simulink model "AOO_group11"  (R2023a)
settings: Solver=FixedStepAuto  StartTime=0.0  StopTime=10.0  FixedStep=1e-3  RelTol=1e-3  EnableMultiTasking=on
undefined symbols (not defined in the file): D10, D11, D2, D4, D5, D8, PTA0, PTA2, PTB23, PTB9, PTD0, PTD2
libraries: frdmk64flib x8
settings Model: ExtModeTrigDuration=5  Creator=faraa  LastModifiedBy=faraa
settings OptimizationCC: EnhancedBackFolding=on  PassReuseOutputArgsAs=Individual arguments  ZeroExternalMemoryAtStartup=off  ZeroInternalMemoryAtStartup=off  MaxStackSize=64  OptimizeBlockOrder=speed  DifferentSizesBufferReuse=on  OptimizationCustomize=off  EfficientTunableParamExpr=on
settings DebuggingCC: ParameterTunabilityLossMsg=error
settings HardwareCC: ProdBitPerPointer=32  ProdBitPerSizeT=32  ProdBitPerPtrDiffT=32  ProdLargestAtomicInteger=Long  ProdLargestAtomicFloat=Double  ProdWordSize=32  ProdHWDeviceType=ARM Compatible->ARM Cortex
settings SFSimCC: MATLABDynamicMemAlloc=off
settings RTWCC: Description=Embedded Coder  SystemTargetFile=ert.tlc  HardwareBoard=NXP FRDM-K64F  TLCOptions="-aInlineSetEventsForThisBaseRateFcn=TLC_FALSE -aSuppressMultiTaskScheduler=TLC_FALSE  -aRateBasedStepFcn=0"  TemplateMakefile=ert_default_tmf  Toolchain=GNU Tools for ARM Embedded Processors
settings CodeAppCC: ForceParamTrailComments=on  IgnoreCustomStorageClasses=off  OperatorAnnotations=on  SimulinkDataObjDesc=on  SFDataObjDesc=on  InsertBlockDesc=on
settings ERTTargetCC: ExtModeTransport=4  ExtModeMexFile=sendToCommService

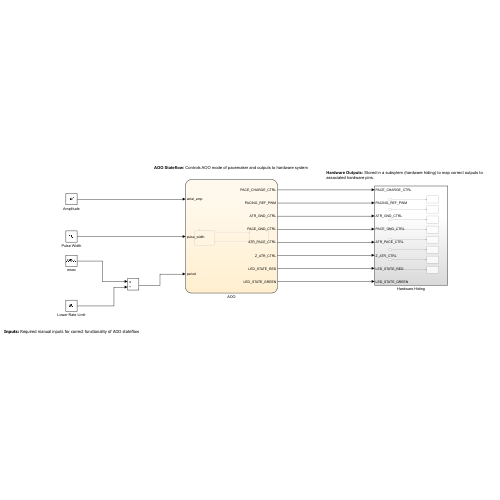
[thumbnail: Simulink's stored preview of the top-level diagram]
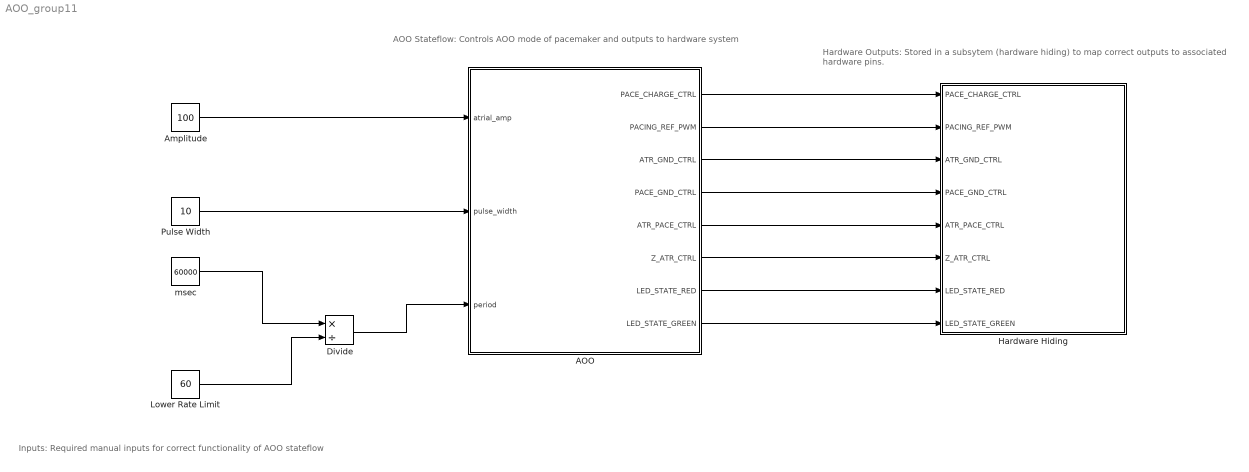
== system AOO_group11 ==
  note: Inputs: Required manual inputs for correct functionality of AOO stateflow
  note: Hardware Outputs: Stored in a subsytem (hardware hiding) to map correct outputs to associated hardware pins.
  note: AOO Stateflow: Controls AOO mode of pacemaker and outputs to hardware system
  AOO : Stateflow chart  TreatAsAtomicUnit=on
      settings: PortSchema="{\"entries\":[{\"content\":{\"sides\":[{\"content\":{\"connectorIds\":[\"In1\",\"In2\",\"In3\"]},\"type\":\"ConnectorPlacement.EquallySpacedRectSide\",\"uuid\":\"95ae3ac6-e5ac-4d1d-8671-90628795223e\"},{\"content\":{\"connectorIds\":[\"Out1\",\"Out2\",\"Out3\",\"Out4\",\"Out5\",\"Out8\",\"Out6\",\"Out7\"],\"side\":\"RIGHT\"},\"type\":\"ConnectorPlacement.EquallySpacedRectSide\",\"uuid\":\"b0ec74bf-e631-4588-a0db-5024556e9f33\"},{\"content\":{\"side\":\"TOP\"},\"type\":\"ConnectorPlacement.EquallySpacedRectSide\",\"uuid\":\"f45d59e1-716f-4ed7-bde8-ed6d2f349a65\"}]},\"type\":\"ConnectorPlacement.EquallySpacedConnector\",\"uuid\":\"a31986a1-9390-4687-9321-72416b41487c\"}],\"packageUris\":[\"http://schema.mathworks.com/mf0/Connector/R2020b\"],\"version\":\"1.0\"}"
  Amplitude : Constant  Value=100
  Divide : Product  Inputs=*/
  Hardware Hiding : Subsystem
  Lower Rate Limit : Constant  Value=60
  Pulse Width : Constant  Value=10
  msec : Constant  Value=60000
  wires:
  Amplitude/1 -> AOO/1(atrial_amp)
  Pulse Width/1 -> AOO/2(pulse_width)
  msec/1 -> Divide/1
  Lower Rate Limit/1 -> Divide/2
  Divide/1 -> AOO/3(period)
  AOO/1(PACE_CHARGE_CTRL) -> Hardware Hiding/1(PACE_CHARGE_CTRL)
  AOO/2(PACING_REF_PWM) -> Hardware Hiding/2(PACING_REF_PWM)
  AOO/3(ATR_GND_CTRL) -> Hardware Hiding/3(ATR_GND_CTRL)
  AOO/4(PACE_GND_CTRL) -> Hardware Hiding/4(PACE_GND_CTRL)
  AOO/5(ATR_PACE_CTRL) -> Hardware Hiding/5(ATR_PACE_CTRL)
  AOO/8(Z_ATR_CTRL) -> Hardware Hiding/6(Z_ATR_CTRL)
  AOO/6(LED_STATE_RED) -> Hardware Hiding/7(LED_STATE_RED)
  AOO/7(LED_STATE_GREEN) -> Hardware Hiding/8(LED_STATE_GREEN)

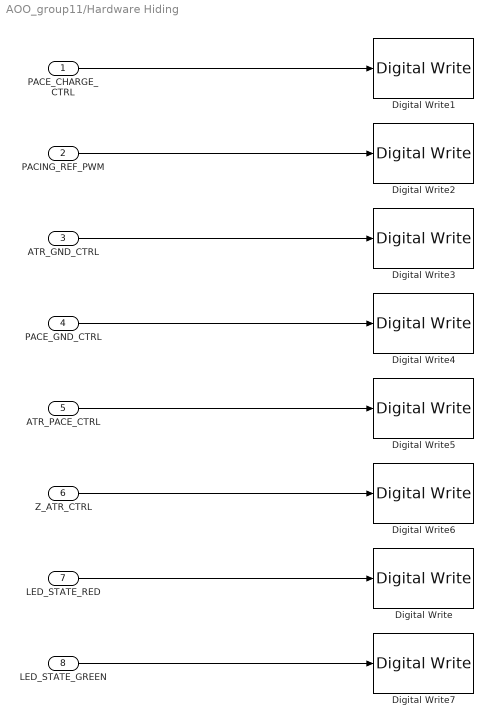
== system AOO_group11/Hardware Hiding ==
  PACE_CHARGE_CTRL : Inport
  PACING_REF_PWM : Inport  Port=2
  ATR_GND_CTRL : Inport  Port=3
  PACE_GND_CTRL : Inport  Port=4
  ATR_PACE_CTRL : Inport  Port=5
  Z_ATR_CTRL : Inport  Port=6
  LED_STATE_RED : Inport  Port=7
  LED_STATE_GREEN : Inport  Port=8
  Digital Write : frdmk64flib/Digital Write  Whichpin=RED_LED
  Digital Write1 : frdmk64flib/Digital Write  Whichpin=PTB9 (D2)
  Digital Write2 : frdmk64flib/Digital Write  Whichpin=PTA2 (D5)
  Digital Write3 : frdmk64flib/Digital Write  Whichpin=PTD2 (D11)
  Digital Write4 : frdmk64flib/Digital Write  Whichpin=PTD0 (D10)
  Digital Write5 : frdmk64flib/Digital Write  Whichpin=PTA0 (D8)
  Digital Write6 : frdmk64flib/Digital Write  Whichpin=PTB23 (D4)
  Digital Write7 : frdmk64flib/Digital Write  Whichpin=GREEN_LED
  wires:
  ATR_PACE_CTRL/1 -> Digital Write5/1
  PACE_GND_CTRL/1 -> Digital Write4/1
  Z_ATR_CTRL/1 -> Digital Write6/1
  PACING_REF_PWM/1 -> Digital Write2/1
  LED_STATE_GREEN/1 -> Digital Write7/1
  LED_STATE_RED/1 -> Digital Write/1
  PACE_CHARGE_CTRL/1 -> Digital Write1/1
  ATR_GND_CTRL/1 -> Digital Write3/1

== stateflow chart AOO_group11/AOO ==
  note: Charging: State to Charge C22 and discharge C21
      | and trigger LED indicators
  note: Pacing: Discharges C22 and charges C21
      | and triggers LED indicators
  state Pacing
    entry:
    PACING_REF_PWM = atrial_amp;
    PACE_CHARGE_CTRL=0;
    ATR_PACE_CTRL= 1;
    ATR_GND_CTRL= 0;
    PACE_GND_CTRL=1;
    Z_ATR_CTRL=0;
    LED_STATE_RED=false;
    LED_STATE_GREEN=true;
  state Charging
    entry:
    PACING_REF_PWM = atrial_amp;
    PACE_CHARGE_CTRL=1;
    ATR_PACE_CTRL= 0;
    ATR_GND_CTRL= 1;
    PACE_GND_CTRL=0;
    Z_ATR_CTRL=0;
    LED_STATE_RED=true;
    LED_STATE_GREEN=false;
  (default) -> Charging
  Charging -> Pacing : [after(period-pulse_width,msec)]
  Pacing -> Charging : [after(pulse_width,msec)]
  data: atrial_amp input; pulse_width input; PACE_CHARGE_CTRL output; PACING_REF_PWM output; ATR_GND_CTRL output; PACE_GND_CTRL output; ATR_PACE_CTRL output; LED_STATE_RED output; LED_STATE_GREEN output; Z_ATR_CTRL output; period input
